simulink model "symulacja_sadowski"  (R2025b)
settings: Solver=VariableStepAuto  StartTime=0.0  StopTime=10.0  MaxStep=1  RelTol=1e-3
values from neighbouring files (symbols this model uses):
  cp = 1000    [skrypt2.m]    (also in skrypt3.m; skrypt4.m)
  Cv1 = cp*pp*Vw1    (= 75000)    [skrypt2.m]    (also in skrypt3.m; skrypt4.m)
  Cv2 = cp*pp*Vw2    (= 75000)    [skrypt2.m]    (also in skrypt3.m; skrypt4.m)
  Fp0 = tab_Fp0(i)    [skrypt2.m]    (also in skrypt3.m = 0.833333333333; skrypt4.m = 0.833333333333)
  K0 = (1-a)*PkN/(Tw1N-Tw2N)    (= 800)    [skrypt2.m]    (also in skrypt3.m; skrypt4.m)
  Ks1 = a*PkN/(Tw1N-TzewN)    (= 150)    [skrypt2.m]    (also in skrypt3.m; skrypt4.m)
  Ks2 = (K0*(Tw1N-Tw2N))/(Tw2N-TzewN)    (= 114.285714286)    [skrypt2.m]    (also in skrypt3.m; skrypt4.m)
  pp = 1.2    [skrypt2.m]    (also in skrypt3.m; skrypt4.m)
  przy_kz = 0    [skrypt2.m]    (also in skrypt3.m = 1; skrypt4.m = 1)
  przy_zew = 2    [skrypt2.m]    (also in skrypt3.m = 0; skrypt4.m = 5)
  przyFp0 = 0    [skrypt2.m]    (also in skrypt3.m; skrypt4.m)
  step_time = 400    [skrypt2.m]    (also in skrypt3.m = 10; skrypt4.m = 100)
  Tkz0 = tab_tk(i)    [skrypt2.m]    (also in skrypt3.m = 30; skrypt4.m = 30)
  Tw1c = ((A*Tkz0 + Ks1*Tzew0)*(K0 + Ks2) + K0*Ks2*Tzew0) / ((A + Ks1 + K0)*(K0 + Ks2) - K0^2)    [skrypt2.m]    (also in skrypt3.m = 20; skrypt4.m = 20)
  Tw2c = ((A + Ks1 + K0)*Ks2*Tzew0 + K0*(A*Tkz0 + Ks1*Tzew0)) / ((A + Ks1 + K0)*(K0 + Ks2) - K0^2)    [skrypt2.m]    (also in skrypt3.m = 15; skrypt4.m = 15)
  Tzew0 = tab_Tzew(i)    [skrypt2.m]    (also in skrypt3.m = -20; skrypt4.m = -20)
settings Model: Creator=mikol  LastModifiedBy=mikol
settings DataIOCC: SignalLogging=off

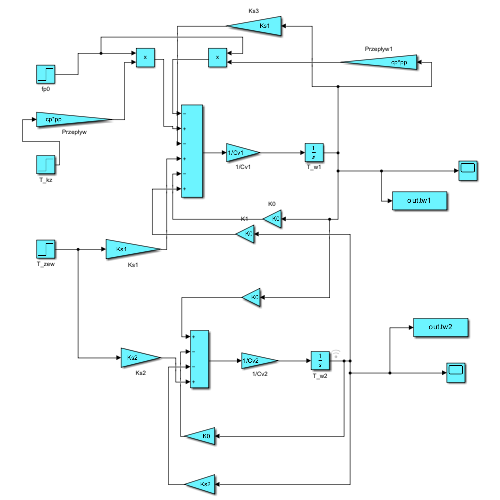
[thumbnail: Simulink's stored preview of the top-level diagram]
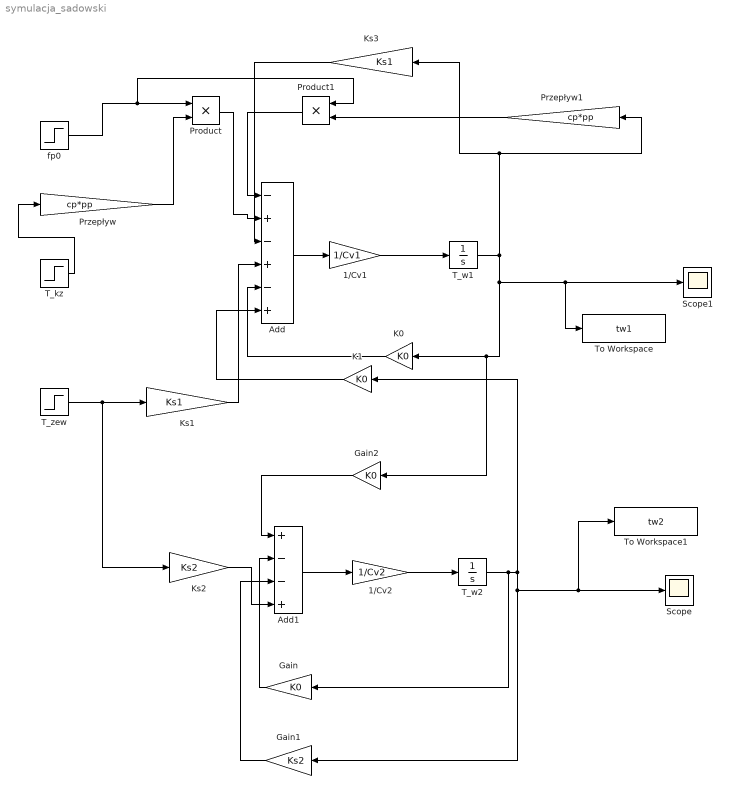
== system symulacja_sadowski ==
  1/Cv1 : Gain  Gain=1/Cv1
  1/Cv2 : Gain  Gain=1/Cv2
  Add : Sum  Inputs=-+-+-+
  Add1 : Sum  Inputs=+--+
  Gain : Gain  Gain=K0
  Gain1 : Gain  Gain=Ks2
  Gain2 : Gain  Gain=K0
  K0 : Gain  Gain=K0
  K1 : Gain  Gain=K0
  Ks1 : Gain  Gain=Ks1
  Ks2 : Gain  Gain=Ks2
  Ks3 : Gain  Gain=Ks1
  Product : Product
  Product1 : Product
  Przepływ : Gain  Gain=cp*pp
  Przepływ1 : Gain  Gain=cp*pp
  Scope : Scope
      settings: ActiveDisplayYMinimum=-8.4999999999999982  ActiveDisplayYMaximum=-6.4999999999999982
  Scope1 : Scope
      settings: ActiveDisplayYMinimum=19.751293239372249  ActiveDisplayYMaximum=22.238360845649765
  T_kz : Step  Time=step_time  Before=Tkz0  After=Tkz0+przy_kz  SampleTime=0
  T_w1 : Integrator  InitialCondition=Tw1c
  T_w2 : Integrator  InitialCondition=Tw2c
  T_zew : Step  Time=step_time  Before=Tzew0  After=Tzew0+przy_zew  SampleTime=0
  To Workspace : ToWorkspace  VariableName=tw1  SampleTime=-1
  To Workspace1 : ToWorkspace  VariableName=tw2  SampleTime=-1
  fp0 : Step  Time=step_time  Before=Fp0  After=Fp0 + przyFp0  SampleTime=0
  wires:
  1/Cv1/1 -> T_w1/1
  T_kz/1 -> Przepływ/1
  Przepływ/1 -> Product/2
  T_w1/1 -> Gain2/1, K0/1, To Workspace/1, Scope1/1, Ks3/1, Przepływ1/1
  T_zew/1 -> Ks2/1, Ks1/1
  Add/1 -> 1/Cv1/1
  Ks3/1 -> Add/3
  Przepływ1/1 -> Product1/2
  K0/1 -> Add/5
  Ks1/1 -> Add/4
  T_w2/1 -> Gain/1, K1/1, Gain1/1, To Workspace1/1, Scope/1
  1/Cv2/1 -> T_w2/1
  K1/1 -> Add/6
  Add1/1 -> 1/Cv2/1
  Ks2/1 -> Add1/4
  Gain/1 -> Add1/2
  Gain1/1 -> Add1/3
  Gain2/1 -> Add1/1
  fp0/1 -> Product1/1, Product/1
  Product/1 -> Add/2
  Product1/1 -> Add/1
